simulink model "fuzzy_PI"  (R2021a)
settings: Solver=VariableStepAuto  StartTime=0.0  StopTime=0.05  RelTol=1e-3
libraries: pid_lib x5, spsPermanentMagnetSynchronousMachineLib x2, spsDCVoltageSourceLib x2, spsUniversalBridgeLib x2, simulink x2, eeGeneralControl x1, spspowerguiLib x1, fuzblock x1
settings Model: Creator=lijingze  LastModifiedBy=lijingze

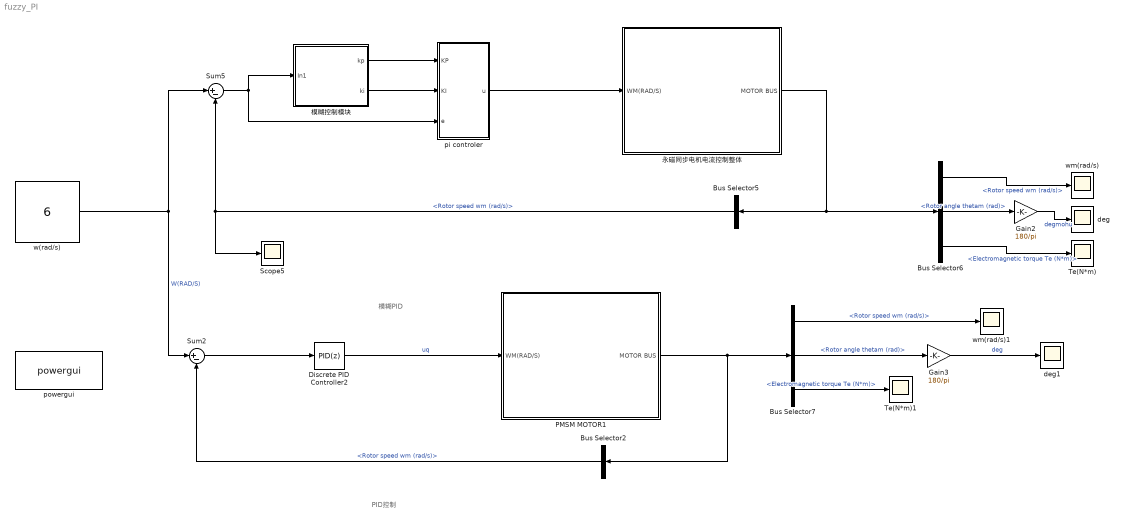
== system fuzzy_PI ==
  note: PID控制
  note: 模糊PID
  Bus Selector2 : BusSelector  OutputSignals=Rotor speed wm (rad/s)
  Bus Selector5 : BusSelector  OutputSignals=Rotor speed wm (rad/s)
  Bus Selector6 : BusSelector  OutputSignals=Rotor speed wm (rad/s),Rotor angle thetam (rad),Electromagnetic torque Te (N*m)
  Bus Selector7 : BusSelector  OutputSignals=Rotor speed wm (rad/s),Rotor angle thetam (rad),Electromagnetic torque Te (N*m)
  Discrete PID Controller2 : pid_lib/PID Controller  Controller=PID  Form=Parallel  TimeDomain=Discrete-time  UseExternalTs=off  SampleTime=-1  IntegratorMethod=Forward Euler  FilterMethod=Forward Euler  ControllerParametersSource=internal  P=40  I=3000  D=0  UseFilter=on  N=100  TunerSelectOption=Transfer Function Based (PID Tuner App)  InitialConditionSource=internal  InitialConditionForIntegrator=0  InitialConditionForFilter=0  DifferentiatorICPrevScaledInput=0  ExternalReset=none  TrackingMode=off  Kt=1  LimitOutput=on  SatLimitsSource=internal  UpperSaturationLimit=100  LowerSaturationLimit=-100  LinearizeAsGain=off  AntiWindupMode=none  Kb=1  POutMin=[]  POutMax=[]  IOutMin=[]  IOutMax=[]  DOutMin=[]  DOutMax=[]  NOutMin=[]  NOutMax=[]  SumOutMin=[]  SumOutMax=[]  SaturationOutMin=[]  SaturationOutMax=[]  PParamMin=[]  PParamMax=[]  IParamMin=[]  IParamMax=[]  DParamMin=[]  DParamMax=[]  NParamMin=[]  NParamMax=[]  KbParamMin=[]  KbParamMax=[]  KtParamMin=[]  KtParamMax=[]  KbOutMin=[]  KbOutMax=[]  KtOutMin=[]  KtOutMax=[]  IntegratorOutMin=[]  IntegratorOutMax=[]  FilterOutMin=[]  FilterOutMax=[]  SumI1OutMin=[]  SumI1OutMax=[]  SumI2OutMin=[]  SumI2OutMax=[]  SumI3OutMin=[]  SumI3OutMax=[]  SumI4OutMin=[]  SumI4OutMax=[]  SumDOutMin=[]  SumDOutMax=[]  DifferentiatorOutMin=[]  DifferentiatorOutMax=[]  FilterDiffOutCoefMin=[]  FilterDiffOutCoefMax=[]  ReciprocalOutMin=[]  ReciprocalOutMax=[]  SumDenOutMin=[]  SumDenOutMax=[]  SumNumOutMin=[]  SumNumOutMax=[]  DivideOutMin=[]  DivideOutMax=[]  UdiffTsProdOutMin=[]  UdiffTsProdOutMax=[]  NTsProdOutMin=[]  NTsProdOutMax=[]  UintegralTsProdOutMin=[]  UintegralTsProdOutMax=[]  UngainTsProdOutMin=[]  UngainTsProdOutMax=[]  IntegratorContinuousStateAttributes=''  IntegratorStateMustResolveToSignalObject=off  IntegratorRTWStateStorageClass=Auto  FilterContinuousStateAttributes=''  FilterStateMustResolveToSignalObject=off  FilterRTWStateStorageClass=Auto  ParallelPVariant=InternalParameters  IdealPVariant=Disabled  IVariant=InternalParameters  DVariant=InternalParameters  IntegratorVariant=Discrete  SatVariant=Enabled  AWVariant=Passthrough  PCopyVariant=Disabled  TRVariant=Disabled  FdbkBlocksVariant=Forward  IdealPFdbkVariant=Disabled  SatFdbkVariant=Disabled  DerivativeFilterVariant=ForwardEulerFilter  NVariant=InternalParameters  NCopyVariant=Disabled  FilterICVariant=InternalICsFilter  IntegratorICVariant=InternalICs  ExternalResetVariant=Disabled  TRSumVariant=Passthrough  SumFdbkVariant=Disabled  SumVariant=Sum_PID  TsampFilterVariant=InternalTs  TsampNgainVariant=Passthrough  TsampIntegralVariant=Passthrough  ExternalSaturationOutDataTypeStr=Inherit: Same as second input
  Gain2 : Gain  Gain=180/pi
  Gain3 : Gain  Gain=180/pi
  PMSM MOTOR1 : Subsystem
  Scope5 : Scope
  Sum2 : Sum  Inputs=|+-
  Sum5 : Sum  Inputs=|+-
  Te(N*m) : Scope
  Te(N*m)1 : Scope
  deg : Scope
  deg1 : Scope
  pi controler : Subsystem
  powergui : spspowerguiLib/powergui  Priority=1  SimulationMode=Discrete  SampleTime=2e-6  frequency=60  Iterations=50  frequencyindice=0  Pbase=100e6  ErrMax=1e-4  UnitsV=kV  UnitsW=MW  buscounter=0  FunctionMessages=off  echomessages=off  EnableUseOfTLC=off  CurrentSourceSwitches=off  DisableSnubberDevices=off  DisableRonSwitches=off  DisableVfSwitches=off  DisplayEquations=off  AutomaticDiscreteSolvers=off  SolverType=Tustin/Backward Euler (TBE)  Interpol=off  ExternalGateDelay=off  methode=off  Ts=100  x0status=blocks  SPID=on  SwTol=0  HookPort=off  NonlinearTolerance=1e-4  nMaxIteration=100  ContinueOnMaxIteration=off  RestoreLinks=warning  ResistiveCurrentMeasurement=off  Frange=[0:2:500]  Ylog=off  Xlog=on  ShowGrid=off  save=off  variable=ZData  structure=0  ZoomFFT=off  StartTime=0.0  cycles=1  DisplayStyle=1  fundamental=60  FreqAxis=off  MaxFrequency=1000  frequencyindicesteady=1  RmsSteady=1  display=off
  w(rad/s) : Constant  Value=6
  wm(rad/s) : Scope
  wm(rad/s)1 : Scope
  模糊控制模块 : Subsystem
  永磁同步电机电流控制整体 : Subsystem
  wires:
  PMSM MOTOR1/1(MOTOR BUS) -> Bus Selector2/1, Bus Selector7/1
  Discrete PID Controller2/1 -> PMSM MOTOR1/1(WM(RAD/S))  "uq"
  永磁同步电机电流控制整体/1(MOTOR BUS) -> Bus Selector5/1, Bus Selector6/1
  pi controler/1(u) -> 永磁同步电机电流控制整体/1(WM(RAD/S))
  Bus Selector6/1 -> wm(rad/s)/1  "<Rotor speed wm (rad/s)>"
  Sum2/1 -> Discrete PID Controller2/1
  Bus Selector6/2 -> Gain2/1  "<Rotor angle thetam (rad)>"
  Bus Selector2/1 -> Sum2/2  "<Rotor speed wm (rad/s)>"
  Bus Selector5/1 -> Scope5/1, Sum5/2  "<Rotor speed wm (rad/s)>"
  Bus Selector6/3 -> Te(N*m)/1  "<Electromagnetic torque Te (N*m)>"
  Gain2/1 -> deg/1  "degmohu"
  Bus Selector7/2 -> Gain3/1  "<Rotor angle thetam (rad)>"
  Sum5/1 -> 模糊控制模块/1(In1), pi controler/3(e)
  w(rad/s)/1 -> Sum2/1, Sum5/1  "W(RAD/S)"
  模糊控制模块/2(ki) -> pi controler/2(KI)
  模糊控制模块/1(kp) -> pi controler/1(KP)
  Bus Selector7/1 -> wm(rad/s)1/1  "<Rotor speed wm (rad/s)>"
  Gain3/1 -> deg1/1  "deg"
  Bus Selector7/3 -> Te(N*m)1/1  "<Electromagnetic torque Te (N*m)>"

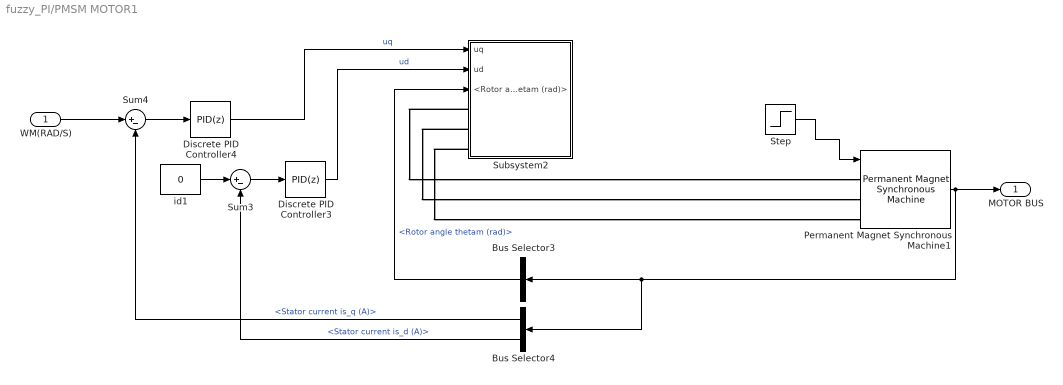
== system fuzzy_PI/PMSM MOTOR1 ==
  WM(RAD/S) : Inport
  Bus Selector3 : BusSelector  OutputSignals=Rotor angle thetam (rad)
  Bus Selector4 : BusSelector  OutputSignals=Stator current is_q (A),Stator current is_d (A)
  Discrete PID Controller3 : pid_lib/PID Controller  Controller=PID  Form=Parallel  TimeDomain=Discrete-time  UseExternalTs=off  SampleTime=-1  IntegratorMethod=Forward Euler  FilterMethod=Forward Euler  ControllerParametersSource=internal  P=50  I=5000  D=0  UseFilter=on  N=100  TunerSelectOption=Transfer Function Based (PID Tuner App)  InitialConditionSource=internal  InitialConditionForIntegrator=0  InitialConditionForFilter=0  DifferentiatorICPrevScaledInput=0  ExternalReset=none  TrackingMode=off  Kt=1  LimitOutput=on  SatLimitsSource=internal  UpperSaturationLimit=100  LowerSaturationLimit=-100  LinearizeAsGain=off  AntiWindupMode=none  Kb=1  POutMin=[]  POutMax=[]  IOutMin=[]  IOutMax=[]  DOutMin=[]  DOutMax=[]  NOutMin=[]  NOutMax=[]  SumOutMin=[]  SumOutMax=[]  SaturationOutMin=[]  SaturationOutMax=[]  PParamMin=[]  PParamMax=[]  IParamMin=[]  IParamMax=[]  DParamMin=[]  DParamMax=[]  NParamMin=[]  NParamMax=[]  KbParamMin=[]  KbParamMax=[]  KtParamMin=[]  KtParamMax=[]  KbOutMin=[]  KbOutMax=[]  KtOutMin=[]  KtOutMax=[]  IntegratorOutMin=[]  IntegratorOutMax=[]  FilterOutMin=[]  FilterOutMax=[]  SumI1OutMin=[]  SumI1OutMax=[]  SumI2OutMin=[]  SumI2OutMax=[]  SumI3OutMin=[]  SumI3OutMax=[]  SumI4OutMin=[]  SumI4OutMax=[]  SumDOutMin=[]  SumDOutMax=[]  DifferentiatorOutMin=[]  DifferentiatorOutMax=[]  FilterDiffOutCoefMin=[]  FilterDiffOutCoefMax=[]  ReciprocalOutMin=[]  ReciprocalOutMax=[]  SumDenOutMin=[]  SumDenOutMax=[]  SumNumOutMin=[]  SumNumOutMax=[]  DivideOutMin=[]  DivideOutMax=[]  UdiffTsProdOutMin=[]  UdiffTsProdOutMax=[]  NTsProdOutMin=[]  NTsProdOutMax=[]  UintegralTsProdOutMin=[]  UintegralTsProdOutMax=[]  UngainTsProdOutMin=[]  UngainTsProdOutMax=[]  IntegratorContinuousStateAttributes=''  IntegratorStateMustResolveToSignalObject=off  IntegratorRTWStateStorageClass=Auto  FilterContinuousStateAttributes=''  FilterStateMustResolveToSignalObject=off  FilterRTWStateStorageClass=Auto  ParallelPVariant=InternalParameters  IdealPVariant=Disabled  IVariant=InternalParameters  DVariant=InternalParameters  IntegratorVariant=Discrete  SatVariant=Enabled  AWVariant=Passthrough  PCopyVariant=Disabled  TRVariant=Disabled  FdbkBlocksVariant=Forward  IdealPFdbkVariant=Disabled  SatFdbkVariant=Disabled  DerivativeFilterVariant=ForwardEulerFilter  NVariant=InternalParameters  NCopyVariant=Disabled  FilterICVariant=InternalICsFilter  IntegratorICVariant=InternalICs  ExternalResetVariant=Disabled  TRSumVariant=Passthrough  SumFdbkVariant=Disabled  SumVariant=Sum_PID  TsampFilterVariant=InternalTs  TsampNgainVariant=Passthrough  TsampIntegralVariant=Passthrough  ExternalSaturationOutDataTypeStr=Inherit: Same as second input
  Discrete PID Controller4 : pid_lib/PID Controller  Controller=PID  Form=Parallel  TimeDomain=Discrete-time  UseExternalTs=off  SampleTime=-1  IntegratorMethod=Forward Euler  FilterMethod=Forward Euler  ControllerParametersSource=internal  P=50  I=5000  D=0  UseFilter=on  N=100  TunerSelectOption=Transfer Function Based (PID Tuner App)  InitialConditionSource=internal  InitialConditionForIntegrator=0  InitialConditionForFilter=0  DifferentiatorICPrevScaledInput=0  ExternalReset=none  TrackingMode=off  Kt=1  LimitOutput=on  SatLimitsSource=internal  UpperSaturationLimit=100  LowerSaturationLimit=-100  LinearizeAsGain=off  AntiWindupMode=none  Kb=1  POutMin=[]  POutMax=[]  IOutMin=[]  IOutMax=[]  DOutMin=[]  DOutMax=[]  NOutMin=[]  NOutMax=[]  SumOutMin=[]  SumOutMax=[]  SaturationOutMin=[]  SaturationOutMax=[]  PParamMin=[]  PParamMax=[]  IParamMin=[]  IParamMax=[]  DParamMin=[]  DParamMax=[]  NParamMin=[]  NParamMax=[]  KbParamMin=[]  KbParamMax=[]  KtParamMin=[]  KtParamMax=[]  KbOutMin=[]  KbOutMax=[]  KtOutMin=[]  KtOutMax=[]  IntegratorOutMin=[]  IntegratorOutMax=[]  FilterOutMin=[]  FilterOutMax=[]  SumI1OutMin=[]  SumI1OutMax=[]  SumI2OutMin=[]  SumI2OutMax=[]  SumI3OutMin=[]  SumI3OutMax=[]  SumI4OutMin=[]  SumI4OutMax=[]  SumDOutMin=[]  SumDOutMax=[]  DifferentiatorOutMin=[]  DifferentiatorOutMax=[]  FilterDiffOutCoefMin=[]  FilterDiffOutCoefMax=[]  ReciprocalOutMin=[]  ReciprocalOutMax=[]  SumDenOutMin=[]  SumDenOutMax=[]  SumNumOutMin=[]  SumNumOutMax=[]  DivideOutMin=[]  DivideOutMax=[]  UdiffTsProdOutMin=[]  UdiffTsProdOutMax=[]  NTsProdOutMin=[]  NTsProdOutMax=[]  UintegralTsProdOutMin=[]  UintegralTsProdOutMax=[]  UngainTsProdOutMin=[]  UngainTsProdOutMax=[]  IntegratorContinuousStateAttributes=''  IntegratorStateMustResolveToSignalObject=off  IntegratorRTWStateStorageClass=Auto  FilterContinuousStateAttributes=''  FilterStateMustResolveToSignalObject=off  FilterRTWStateStorageClass=Auto  ParallelPVariant=InternalParameters  IdealPVariant=Disabled  IVariant=InternalParameters  DVariant=InternalParameters  IntegratorVariant=Discrete  SatVariant=Enabled  AWVariant=Passthrough  PCopyVariant=Disabled  TRVariant=Disabled  FdbkBlocksVariant=Forward  IdealPFdbkVariant=Disabled  SatFdbkVariant=Disabled  DerivativeFilterVariant=ForwardEulerFilter  NVariant=InternalParameters  NCopyVariant=Disabled  FilterICVariant=InternalICsFilter  IntegratorICVariant=InternalICs  ExternalResetVariant=Disabled  TRSumVariant=Passthrough  SumFdbkVariant=Disabled  SumVariant=Sum_PID  TsampFilterVariant=InternalTs  TsampNgainVariant=Passthrough  TsampIntegralVariant=Passthrough  ExternalSaturationOutDataTypeStr=Inherit: Same as second input
  Permanent Magnet Synchronous Machine1 : spsPermanentMagnetSynchronousMachineLib/Permanent Magnet Synchronous Machine  NbPhases=3  FluxDistribution=Sinusoidal  RotorType=Round  MechanicalLoad=Torque Tm  PresetModel=No  ShowDetailedParameters=on  MeasurementBus=off  Resistance=0.0485  Inductance=8.5e-3  dqInductances=[8.5e-3,8.5e-3]  La=0.000395  MachineConstant=Flux linkage established by magnets (V.s)  Flux=0.1194  VoltageCst=21.6568  TorqueCst=0.1791  Flat=120  Mechanical=[0.0027 0.04924 1 0]  PolePairs=4  InitialConditions=[0,0, 0,0]  InitialConditions5ph=[0 0 0 0 0 0]  RefAngle=Aligned with phase A axis (original Park)  IterativeDiscreteModel=Trapezoidal non iterative  TsBlock=-1  TsPowergui=0
  Step : Step  Time=0.025  Before=5  After=10  SampleTime=0.025
  Subsystem2 : Subsystem
  Sum3 : Sum  Inputs=|+-
  Sum4 : Sum  Inputs=|+-
  id1 : Constant  Value=0
  MOTOR BUS : Outport
  wires:
  Discrete PID Controller3/1 -> Subsystem2/2(ud)  "ud"
  Bus Selector3/1 -> Subsystem2/3(<Rotor angle thetam (rad)>)  "<Rotor angle thetam (rad)>"
  Sum4/1 -> Discrete PID Controller4/1
  Permanent Magnet Synchronous Machine1/1 -> Bus Selector4/1, Bus Selector3/1, MOTOR BUS/1
  id1/1 -> Sum3/1
  Bus Selector4/2 -> Sum3/2  "<Stator current is_d (A)>"
  Discrete PID Controller4/1 -> Subsystem2/1(uq)  "uq"
  Sum3/1 -> Discrete PID Controller3/1
  Bus Selector4/1 -> Sum4/2  "<Stator current is_q (A)>"
  Step/1 -> Permanent Magnet Synchronous Machine1/1
  WM(RAD/S)/1 -> Sum4/1
  connections:
  Subsystem2/LConn3 -- Permanent Magnet Synchronous Machine1/LConn3
  Subsystem2/LConn2 -- Permanent Magnet Synchronous Machine1/LConn2
  Subsystem2/LConn1 -- Permanent Magnet Synchronous Machine1/LConn1

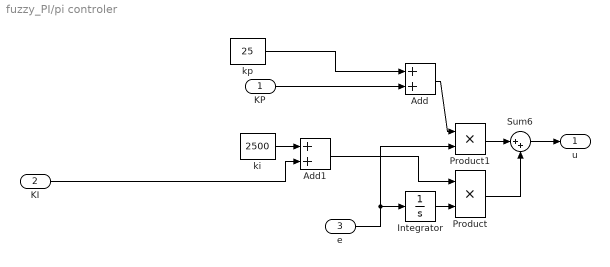
== system fuzzy_PI/pi controler ==
  KP : Inport
  KI : Inport  Port=2
  e : Inport  Port=3
  Add : Sum
  Add1 : Sum
  Integrator : Integrator
  Product : Product
  Product1 : Product
  Sum6 : Sum  Inputs=|++
  ki : Constant  Value=2500
  kp : Constant  Value=25
  u : Outport
  wires:
  Integrator/1 -> Product/2
  e/1 -> Product1/2, Integrator/1
  Product1/1 -> Sum6/1
  Product/1 -> Sum6/2
  Sum6/1 -> u/1
  KP/1 -> Add/2
  kp/1 -> Add/1
  Add/1 -> Product1/1
  ki/1 -> Add1/1
  KI/1 -> Add1/2
  Add1/1 -> Product/1

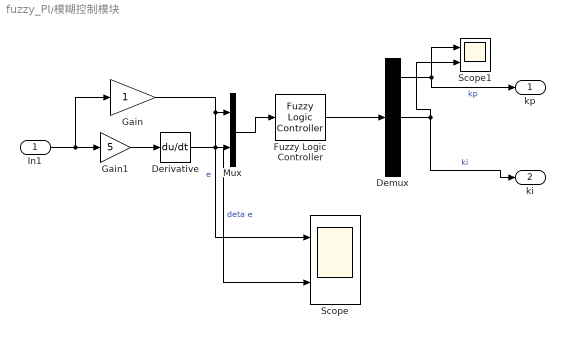
== system fuzzy_PI/模糊控制模块 ==
  In1 : Inport
  Demux : Demux  Outputs=3
  Derivative : Derivative
  Fuzzy Logic Controller : fuzblock/Fuzzy Logic  Controller  FIS=fuzzy_pid  OutputSampleNumber=101  DataType=double  FuzzifiedInputs=off  RuleFiringStrengths=off  RuleOutputs=off  AggregatedOutputs=off  SimulateUsing=Code generation  OutOfRangeInputValueMessage=warning  NoRuleFiredMessage=warning  EmptyOutputFuzzySetMessage=warning
  Gain : Gain
  Gain1 : Gain  Gain=5
  Mux : Mux  Inputs=2
  Scope : Scope  NumInputPorts=2
  Scope1 : Scope  NumInputPorts=2
  kp : Outport
  ki : Outport  Port=2
  wires:
  In1/1 -> Gain/1, Gain1/1
  Mux/1 -> Fuzzy Logic Controller/1
  Gain/1 -> Scope/1, Mux/1  "e"
  Gain1/1 -> Derivative/1
  Derivative/1 -> Scope/2, Mux/2  "deta e"
  Fuzzy Logic Controller/1 -> Demux/1
  Demux/1 -> kp/1, Scope1/1  "kp"
  Demux/2 -> ki/1, Scope1/2  "ki"

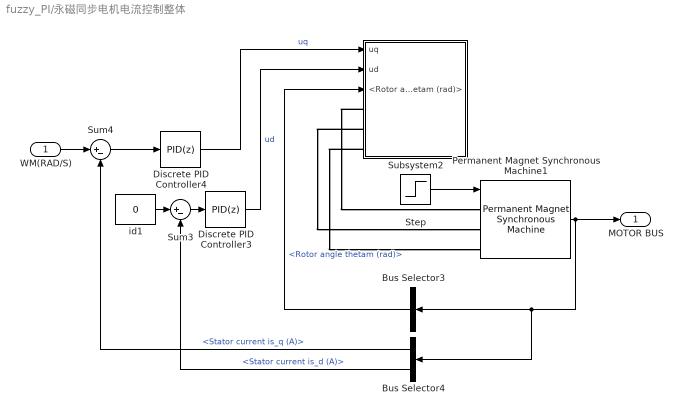
== system fuzzy_PI/永磁同步电机电流控制整体 ==
  WM(RAD/S) : Inport
  Bus Selector3 : BusSelector  OutputSignals=Rotor angle thetam (rad)
  Bus Selector4 : BusSelector  OutputSignals=Stator current is_q (A),Stator current is_d (A)
  Discrete PID Controller3 : pid_lib/PID Controller  Controller=PID  Form=Parallel  TimeDomain=Discrete-time  UseExternalTs=off  SampleTime=-1  IntegratorMethod=Forward Euler  FilterMethod=Forward Euler  ControllerParametersSource=internal  P=50  I=5000  D=0  UseFilter=on  N=100  TunerSelectOption=Transfer Function Based (PID Tuner App)  InitialConditionSource=internal  InitialConditionForIntegrator=0  InitialConditionForFilter=0  DifferentiatorICPrevScaledInput=0  ExternalReset=none  TrackingMode=off  Kt=1  LimitOutput=on  SatLimitsSource=internal  UpperSaturationLimit=100  LowerSaturationLimit=-100  LinearizeAsGain=off  AntiWindupMode=none  Kb=1  POutMin=[]  POutMax=[]  IOutMin=[]  IOutMax=[]  DOutMin=[]  DOutMax=[]  NOutMin=[]  NOutMax=[]  SumOutMin=[]  SumOutMax=[]  SaturationOutMin=[]  SaturationOutMax=[]  PParamMin=[]  PParamMax=[]  IParamMin=[]  IParamMax=[]  DParamMin=[]  DParamMax=[]  NParamMin=[]  NParamMax=[]  KbParamMin=[]  KbParamMax=[]  KtParamMin=[]  KtParamMax=[]  KbOutMin=[]  KbOutMax=[]  KtOutMin=[]  KtOutMax=[]  IntegratorOutMin=[]  IntegratorOutMax=[]  FilterOutMin=[]  FilterOutMax=[]  SumI1OutMin=[]  SumI1OutMax=[]  SumI2OutMin=[]  SumI2OutMax=[]  SumI3OutMin=[]  SumI3OutMax=[]  SumI4OutMin=[]  SumI4OutMax=[]  SumDOutMin=[]  SumDOutMax=[]  DifferentiatorOutMin=[]  DifferentiatorOutMax=[]  FilterDiffOutCoefMin=[]  FilterDiffOutCoefMax=[]  ReciprocalOutMin=[]  ReciprocalOutMax=[]  SumDenOutMin=[]  SumDenOutMax=[]  SumNumOutMin=[]  SumNumOutMax=[]  DivideOutMin=[]  DivideOutMax=[]  UdiffTsProdOutMin=[]  UdiffTsProdOutMax=[]  NTsProdOutMin=[]  NTsProdOutMax=[]  UintegralTsProdOutMin=[]  UintegralTsProdOutMax=[]  UngainTsProdOutMin=[]  UngainTsProdOutMax=[]  IntegratorContinuousStateAttributes=''  IntegratorStateMustResolveToSignalObject=off  IntegratorRTWStateStorageClass=Auto  FilterContinuousStateAttributes=''  FilterStateMustResolveToSignalObject=off  FilterRTWStateStorageClass=Auto  ParallelPVariant=InternalParameters  IdealPVariant=Disabled  IVariant=InternalParameters  DVariant=InternalParameters  IntegratorVariant=Discrete  SatVariant=Enabled  AWVariant=Passthrough  PCopyVariant=Disabled  TRVariant=Disabled  FdbkBlocksVariant=Forward  IdealPFdbkVariant=Disabled  SatFdbkVariant=Disabled  DerivativeFilterVariant=ForwardEulerFilter  NVariant=InternalParameters  NCopyVariant=Disabled  FilterICVariant=InternalICsFilter  IntegratorICVariant=InternalICs  ExternalResetVariant=Disabled  TRSumVariant=Passthrough  SumFdbkVariant=Disabled  SumVariant=Sum_PID  TsampFilterVariant=InternalTs  TsampNgainVariant=Passthrough  TsampIntegralVariant=Passthrough  ExternalSaturationOutDataTypeStr=Inherit: Same as second input
  Discrete PID Controller4 : pid_lib/PID Controller  Controller=PID  Form=Parallel  TimeDomain=Discrete-time  UseExternalTs=off  SampleTime=-1  IntegratorMethod=Forward Euler  FilterMethod=Forward Euler  ControllerParametersSource=internal  P=50  I=5000  D=0  UseFilter=on  N=100  TunerSelectOption=Transfer Function Based (PID Tuner App)  InitialConditionSource=internal  InitialConditionForIntegrator=0  InitialConditionForFilter=0  DifferentiatorICPrevScaledInput=0  ExternalReset=none  TrackingMode=off  Kt=1  LimitOutput=on  SatLimitsSource=internal  UpperSaturationLimit=100  LowerSaturationLimit=-100  LinearizeAsGain=off  AntiWindupMode=none  Kb=1  POutMin=[]  POutMax=[]  IOutMin=[]  IOutMax=[]  DOutMin=[]  DOutMax=[]  NOutMin=[]  NOutMax=[]  SumOutMin=[]  SumOutMax=[]  SaturationOutMin=[]  SaturationOutMax=[]  PParamMin=[]  PParamMax=[]  IParamMin=[]  IParamMax=[]  DParamMin=[]  DParamMax=[]  NParamMin=[]  NParamMax=[]  KbParamMin=[]  KbParamMax=[]  KtParamMin=[]  KtParamMax=[]  KbOutMin=[]  KbOutMax=[]  KtOutMin=[]  KtOutMax=[]  IntegratorOutMin=[]  IntegratorOutMax=[]  FilterOutMin=[]  FilterOutMax=[]  SumI1OutMin=[]  SumI1OutMax=[]  SumI2OutMin=[]  SumI2OutMax=[]  SumI3OutMin=[]  SumI3OutMax=[]  SumI4OutMin=[]  SumI4OutMax=[]  SumDOutMin=[]  SumDOutMax=[]  DifferentiatorOutMin=[]  DifferentiatorOutMax=[]  FilterDiffOutCoefMin=[]  FilterDiffOutCoefMax=[]  ReciprocalOutMin=[]  ReciprocalOutMax=[]  SumDenOutMin=[]  SumDenOutMax=[]  SumNumOutMin=[]  SumNumOutMax=[]  DivideOutMin=[]  DivideOutMax=[]  UdiffTsProdOutMin=[]  UdiffTsProdOutMax=[]  NTsProdOutMin=[]  NTsProdOutMax=[]  UintegralTsProdOutMin=[]  UintegralTsProdOutMax=[]  UngainTsProdOutMin=[]  UngainTsProdOutMax=[]  IntegratorContinuousStateAttributes=''  IntegratorStateMustResolveToSignalObject=off  IntegratorRTWStateStorageClass=Auto  FilterContinuousStateAttributes=''  FilterStateMustResolveToSignalObject=off  FilterRTWStateStorageClass=Auto  ParallelPVariant=InternalParameters  IdealPVariant=Disabled  IVariant=InternalParameters  DVariant=InternalParameters  IntegratorVariant=Discrete  SatVariant=Enabled  AWVariant=Passthrough  PCopyVariant=Disabled  TRVariant=Disabled  FdbkBlocksVariant=Forward  IdealPFdbkVariant=Disabled  SatFdbkVariant=Disabled  DerivativeFilterVariant=ForwardEulerFilter  NVariant=InternalParameters  NCopyVariant=Disabled  FilterICVariant=InternalICsFilter  IntegratorICVariant=InternalICs  ExternalResetVariant=Disabled  TRSumVariant=Passthrough  SumFdbkVariant=Disabled  SumVariant=Sum_PID  TsampFilterVariant=InternalTs  TsampNgainVariant=Passthrough  TsampIntegralVariant=Passthrough  ExternalSaturationOutDataTypeStr=Inherit: Same as second input
  Permanent Magnet Synchronous Machine1 : spsPermanentMagnetSynchronousMachineLib/Permanent Magnet Synchronous Machine  NbPhases=3  FluxDistribution=Sinusoidal  RotorType=Round  MechanicalLoad=Torque Tm  PresetModel=No  ShowDetailedParameters=on  MeasurementBus=off  Resistance=0.0485  Inductance=8.5e-3  dqInductances=[8.5e-3,8.5e-3]  La=0.000395  MachineConstant=Flux linkage established by magnets (V.s)  Flux=0.1194  VoltageCst=21.6568  TorqueCst=0.1791  Flat=120  Mechanical=[0.0027 0.04924 1 0]  PolePairs=4  InitialConditions=[0,0, 0,0]  InitialConditions5ph=[0 0 0 0 0 0]  RefAngle=Aligned with phase A axis (original Park)  IterativeDiscreteModel=Trapezoidal non iterative  TsBlock=-1  TsPowergui=0
  Step : Step  Time=0.025  Before=5  After=10  SampleTime=0.025
  Subsystem2 : Subsystem
  Sum3 : Sum  Inputs=|+-
  Sum4 : Sum  Inputs=|+-
  id1 : Constant  Value=0
  MOTOR BUS : Outport
  wires:
  Discrete PID Controller3/1 -> Subsystem2/2(ud)  "ud"
  Bus Selector3/1 -> Subsystem2/3(<Rotor angle thetam (rad)>)  "<Rotor angle thetam (rad)>"
  Sum4/1 -> Discrete PID Controller4/1
  Permanent Magnet Synchronous Machine1/1 -> Bus Selector4/1, Bus Selector3/1, MOTOR BUS/1
  id1/1 -> Sum3/1
  Bus Selector4/2 -> Sum3/2  "<Stator current is_d (A)>"
  Discrete PID Controller4/1 -> Subsystem2/1(uq)  "uq"
  Sum3/1 -> Discrete PID Controller3/1
  Bus Selector4/1 -> Sum4/2  "<Stator current is_q (A)>"
  WM(RAD/S)/1 -> Sum4/1
  Step/1 -> Permanent Magnet Synchronous Machine1/1
  connections:
  Subsystem2/LConn3 -- Permanent Magnet Synchronous Machine1/LConn3
  Subsystem2/LConn2 -- Permanent Magnet Synchronous Machine1/LConn2
  Subsystem2/LConn1 -- Permanent Magnet Synchronous Machine1/LConn1

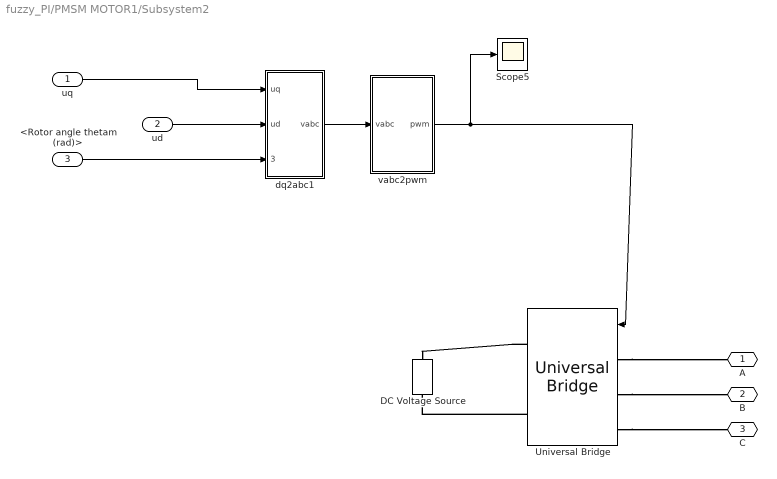
== system fuzzy_PI/PMSM MOTOR1/Subsystem2 ==
  uq : Inport
  ud : Inport  Port=2
  <Rotor angle thetam (rad)> : Inport  Port=3
  DC Voltage Source : spsDCVoltageSourceLib/DC Voltage Source  Amplitude=100  Measurements=None
  Scope5 : Scope
  Universal Bridge : spsUniversalBridgeLib/Universal Bridge  Arms=3  SnubberResistance=1e5  SnubberCapacitance=inf  Device=MOSFET / Diodes  Ron=1e-3  Lon=0  ForwardVoltages="[  0  0  ]"  ForwardVoltage=0  GTOparameters=[ 10e-6 , 20e-6 ]  IGBTparameters=[ 1e-6 , 2e-6 ]  Measurements=None  Measurements_2=None  converterType=Rectifier
  dq2abc1 : Subsystem
  vabc2pwm : Subsystem
  A : PMIOPort  Side=Left
  B : PMIOPort  Port=2  Side=Left
  C : PMIOPort  Port=3  Side=Left
  wires:
  uq/1 -> dq2abc1/1(uq)
  <Rotor angle thetam (rad)>/1 -> dq2abc1/3(" theta")
  vabc2pwm/1(pwm) -> Scope5/1, Universal Bridge/1
  ud/1 -> dq2abc1/2(ud)
  dq2abc1/1(vabc) -> vabc2pwm/1(vabc)
  connections:
  Universal Bridge/LConn2 -- B/RConn1
  Universal Bridge/RConn1 -- DC Voltage Source/RConn1
  Universal Bridge/RConn2 -- DC Voltage Source/LConn1
  Universal Bridge/LConn1 -- A/RConn1
  Universal Bridge/LConn3 -- C/RConn1

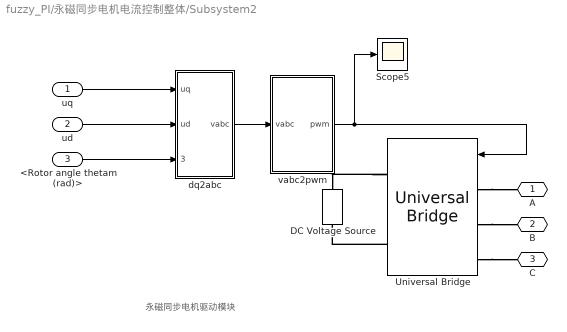
== system fuzzy_PI/永磁同步电机电流控制整体/Subsystem2 ==
  note: 永磁同步电机驱动模块
  uq : Inport
  ud : Inport  Port=2
  <Rotor angle thetam (rad)> : Inport  Port=3
  DC Voltage Source : spsDCVoltageSourceLib/DC Voltage Source  Amplitude=100  Measurements=None
  Scope5 : Scope
  Universal Bridge : spsUniversalBridgeLib/Universal Bridge  Arms=3  SnubberResistance=1e5  SnubberCapacitance=inf  Device=MOSFET / Diodes  Ron=1e-3  Lon=0  ForwardVoltages="[  0  0  ]"  ForwardVoltage=0  GTOparameters=[ 10e-6 , 20e-6 ]  IGBTparameters=[ 1e-6 , 2e-6 ]  Measurements=None  Measurements_2=None  converterType=Rectifier
  dq2abc : Subsystem
  vabc2pwm : Subsystem
  A : PMIOPort  Side=Left
  B : PMIOPort  Port=2  Side=Left
  C : PMIOPort  Port=3  Side=Left
  wires:
  uq/1 -> dq2abc/1(uq)
  <Rotor angle thetam (rad)>/1 -> dq2abc/3(" theta")
  vabc2pwm/1(pwm) -> Universal Bridge/1, Scope5/1
  ud/1 -> dq2abc/2(ud)
  dq2abc/1(vabc) -> vabc2pwm/1(vabc)
  connections:
  Universal Bridge/LConn2 -- B/RConn1
  Universal Bridge/RConn1 -- DC Voltage Source/RConn1
  Universal Bridge/RConn2 -- DC Voltage Source/LConn1
  Universal Bridge/LConn1 -- A/RConn1
  Universal Bridge/LConn3 -- C/RConn1

== system fuzzy_PI/PMSM MOTOR1/Subsystem2/dq2abc1 ==
  uq : Inport
  ud : Inport  Port=2
  " theta" : Inport  Port=3
  Mux : Mux  Inputs=3
  Scope1 : Scope
  Subsystem : Subsystem
  Subsystem1 : Subsystem
  Subsystem2 : Subsystem
  vabc : Outport
  wires:
  ud/1 -> Subsystem/2(ud), Subsystem2/2(ud), Subsystem1/2(ud)
  uq/1 -> Subsystem2/1(uq), Subsystem1/1(uq), Subsystem/1(uq)
  " theta"/1 -> Subsystem2/3(" theta"), Subsystem1/3(" theta"), Subsystem/3(" theta")
  Subsystem/1(ua) -> Mux/1
  Mux/1 -> Scope1/1, vabc/1
  Subsystem2/1(ua) -> Mux/3
  Subsystem1/1(ua) -> Mux/2

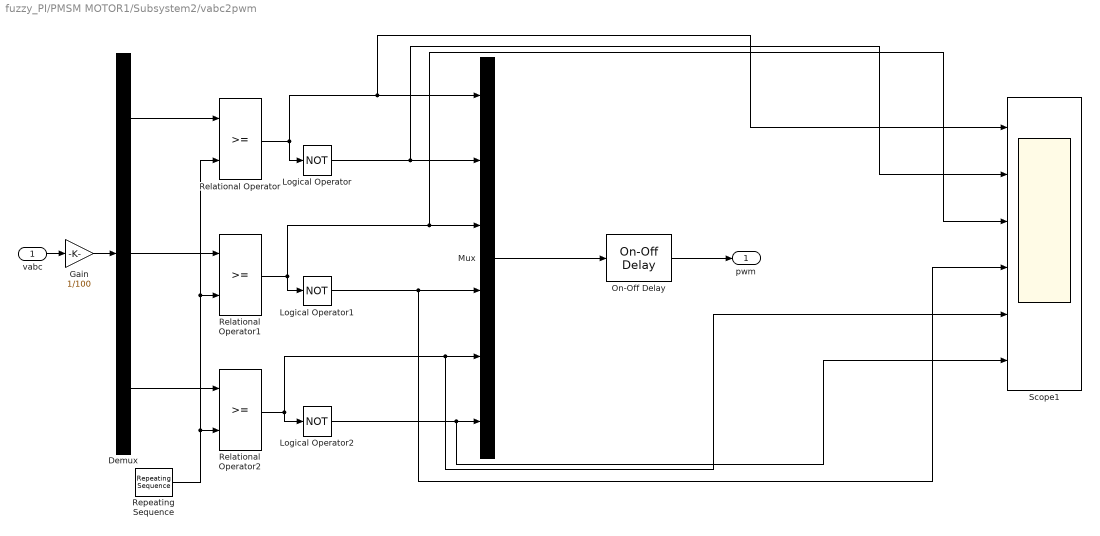
== system fuzzy_PI/PMSM MOTOR1/Subsystem2/vabc2pwm ==
  vabc : Inport
  Demux : Demux  Outputs=3
  Gain : Gain  Gain=1/100
  Logical Operator : Logic  Operator=NOT  AllPortsSameDT=off  OutDataTypeStr=boolean
  Logical Operator1 : Logic  Operator=NOT  AllPortsSameDT=off  OutDataTypeStr=boolean
  Logical Operator2 : Logic  Operator=NOT  AllPortsSameDT=off  OutDataTypeStr=boolean
  Mux : Mux  Inputs=6
  On-Off Delay : eeGeneralControl/On-Off Delay  LabelModeActiveChoice=Discrete  Td_on=2e-6  Td_off=0  IC=0  Ts=2e-6
      settings: SourceProductBaseCode=PS
  Relational Operator : RelationalOperator  OutDataTypeStr=boolean  RndMeth=Simplest
  Relational Operator1 : RelationalOperator  OutDataTypeStr=boolean  RndMeth=Simplest
  Relational Operator2 : RelationalOperator  OutDataTypeStr=boolean  RndMeth=Simplest
  Repeating Sequence : simulink/Sources/Repeating Sequence  rep_seq_t=[0 0.0001]  rep_seq_y=[-1 1]
  Scope1 : Scope  NumInputPorts=6
  pwm : Outport
  wires:
  Repeating Sequence/1 -> Relational Operator/2, Relational Operator1/2, Relational Operator2/2
  Demux/1 -> Relational Operator/1
  Logical Operator/1 -> Scope1/2, Mux/2
  Relational Operator/1 -> Scope1/1, Mux/1, Logical Operator/1
  Demux/3 -> Relational Operator2/1
  Demux/2 -> Relational Operator1/1
  Relational Operator1/1 -> Scope1/3, Mux/3, Logical Operator1/1
  Relational Operator2/1 -> Scope1/5, Mux/5, Logical Operator2/1
  Logical Operator2/1 -> Scope1/6, Mux/6
  Logical Operator1/1 -> Scope1/4, Mux/4
  vabc/1 -> Gain/1
  Gain/1 -> Demux/1
  Mux/1 -> On-Off Delay/1
  On-Off Delay/1 -> pwm/1

== system fuzzy_PI/永磁同步电机电流控制整体/Subsystem2/dq2abc ==
  uq : Inport
  ud : Inport  Port=2
  " theta" : Inport  Port=3
  Mux : Mux  Inputs=3
  Scope1 : Scope
  Subsystem : Subsystem
  Subsystem1 : Subsystem
  Subsystem2 : Subsystem
  vabc : Outport
  wires:
  ud/1 -> Subsystem/2(ud), Subsystem2/2(ud), Subsystem1/2(ud)
  uq/1 -> Subsystem2/1(uq), Subsystem1/1(uq), Subsystem/1(uq)
  " theta"/1 -> Subsystem2/3(" theta"), Subsystem1/3(" theta"), Subsystem/3(" theta")
  Subsystem/1(ua) -> Mux/1
  Mux/1 -> Scope1/1, vabc/1
  Subsystem2/1(ua) -> Mux/3
  Subsystem1/1(ua) -> Mux/2

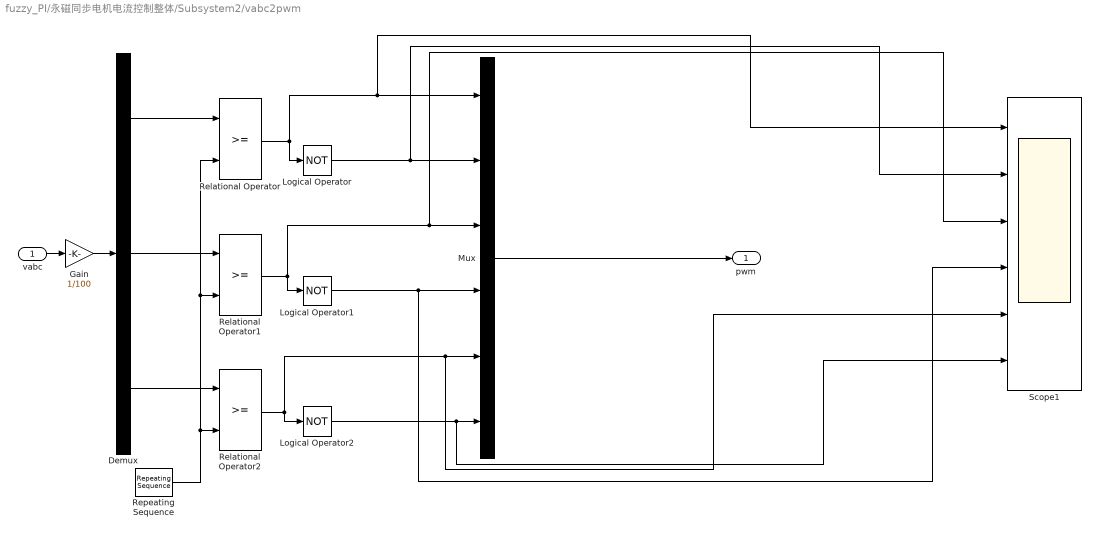
== system fuzzy_PI/永磁同步电机电流控制整体/Subsystem2/vabc2pwm ==
  vabc : Inport
  Demux : Demux  Outputs=3
  Gain : Gain  Gain=1/100
  Logical Operator : Logic  Operator=NOT  AllPortsSameDT=off  OutDataTypeStr=boolean
  Logical Operator1 : Logic  Operator=NOT  AllPortsSameDT=off  OutDataTypeStr=boolean
  Logical Operator2 : Logic  Operator=NOT  AllPortsSameDT=off  OutDataTypeStr=boolean
  Mux : Mux  Inputs=6
  Relational Operator : RelationalOperator  OutDataTypeStr=boolean  RndMeth=Simplest
  Relational Operator1 : RelationalOperator  OutDataTypeStr=boolean  RndMeth=Simplest
  Relational Operator2 : RelationalOperator  OutDataTypeStr=boolean  RndMeth=Simplest
  Repeating Sequence : simulink/Sources/Repeating Sequence  rep_seq_t=[0 0.0001]  rep_seq_y=[-1 1]
  Scope1 : Scope  NumInputPorts=6
  pwm : Outport
  wires:
  Repeating Sequence/1 -> Relational Operator/2, Relational Operator1/2, Relational Operator2/2
  Demux/1 -> Relational Operator/1
  Logical Operator/1 -> Scope1/2, Mux/2
  Relational Operator/1 -> Scope1/1, Mux/1, Logical Operator/1
  Demux/3 -> Relational Operator2/1
  Demux/2 -> Relational Operator1/1
  Relational Operator1/1 -> Scope1/3, Mux/3, Logical Operator1/1
  Relational Operator2/1 -> Scope1/5, Mux/5, Logical Operator2/1
  Logical Operator2/1 -> Scope1/6, Mux/6
  Logical Operator1/1 -> Scope1/4, Mux/4
  vabc/1 -> Gain/1
  Gain/1 -> Demux/1
  Mux/1 -> pwm/1

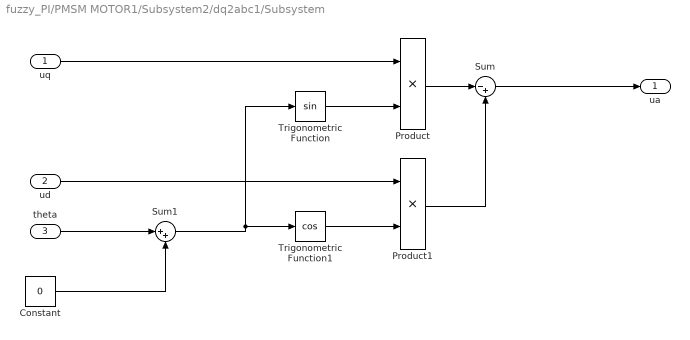
== system fuzzy_PI/PMSM MOTOR1/Subsystem2/dq2abc1/Subsystem ==
  uq : Inport
  ud : Inport  Port=2
  " theta" : Inport  Port=3
  Constant : Constant  Value=0
  Product : Product
  Product1 : Product
  Sum : Sum  Inputs=|-+
  Sum1 : Sum  Inputs=|++
  Trigonometric Function : Trigonometry
  Trigonometric Function1 : Trigonometry  Operator=cos
  ua : Outport
  wires:
  Sum/1 -> ua/1
  Product1/1 -> Sum/2
  ud/1 -> Product1/1
  uq/1 -> Product/1
  Trigonometric Function/1 -> Product/2
  Product/1 -> Sum/1
  Trigonometric Function1/1 -> Product1/2
  " theta"/1 -> Sum1/1
  Sum1/1 -> Trigonometric Function/1, Trigonometric Function1/1
  Constant/1 -> Sum1/2

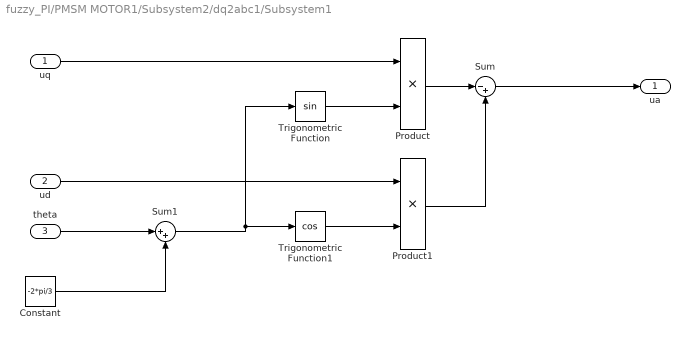
== system fuzzy_PI/PMSM MOTOR1/Subsystem2/dq2abc1/Subsystem1 ==
  uq : Inport
  ud : Inport  Port=2
  " theta" : Inport  Port=3
  Constant : Constant  Value=-2*pi/3
  Product : Product
  Product1 : Product
  Sum : Sum  Inputs=|-+
  Sum1 : Sum  Inputs=|++
  Trigonometric Function : Trigonometry
  Trigonometric Function1 : Trigonometry  Operator=cos
  ua : Outport
  wires:
  Sum/1 -> ua/1
  Product1/1 -> Sum/2
  ud/1 -> Product1/1
  uq/1 -> Product/1
  Trigonometric Function/1 -> Product/2
  Product/1 -> Sum/1
  Trigonometric Function1/1 -> Product1/2
  " theta"/1 -> Sum1/1
  Sum1/1 -> Trigonometric Function/1, Trigonometric Function1/1
  Constant/1 -> Sum1/2

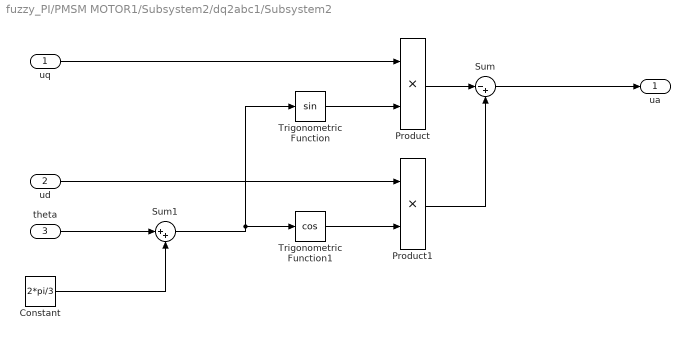
== system fuzzy_PI/PMSM MOTOR1/Subsystem2/dq2abc1/Subsystem2 ==
  uq : Inport
  ud : Inport  Port=2
  " theta" : Inport  Port=3
  Constant : Constant  Value=2*pi/3
  Product : Product
  Product1 : Product
  Sum : Sum  Inputs=|-+
  Sum1 : Sum  Inputs=|++
  Trigonometric Function : Trigonometry
  Trigonometric Function1 : Trigonometry  Operator=cos
  ua : Outport
  wires:
  Sum/1 -> ua/1
  Product1/1 -> Sum/2
  ud/1 -> Product1/1
  uq/1 -> Product/1
  Trigonometric Function/1 -> Product/2
  Product/1 -> Sum/1
  Trigonometric Function1/1 -> Product1/2
  " theta"/1 -> Sum1/1
  Sum1/1 -> Trigonometric Function/1, Trigonometric Function1/1
  Constant/1 -> Sum1/2

== system fuzzy_PI/永磁同步电机电流控制整体/Subsystem2/dq2abc/Subsystem ==
  uq : Inport
  ud : Inport  Port=2
  " theta" : Inport  Port=3
  Constant : Constant  Value=0
  Product : Product
  Product1 : Product
  Sum : Sum  Inputs=|-+
  Sum1 : Sum  Inputs=|++
  Trigonometric Function : Trigonometry
  Trigonometric Function1 : Trigonometry  Operator=cos
  ua : Outport
  wires:
  Sum/1 -> ua/1
  Product1/1 -> Sum/2
  ud/1 -> Product1/1
  uq/1 -> Product/1
  Trigonometric Function/1 -> Product/2
  Product/1 -> Sum/1
  Trigonometric Function1/1 -> Product1/2
  " theta"/1 -> Sum1/1
  Sum1/1 -> Trigonometric Function/1, Trigonometric Function1/1
  Constant/1 -> Sum1/2

== system fuzzy_PI/永磁同步电机电流控制整体/Subsystem2/dq2abc/Subsystem1 ==
  uq : Inport
  ud : Inport  Port=2
  " theta" : Inport  Port=3
  Constant : Constant  Value=-2*pi/3
  Product : Product
  Product1 : Product
  Sum : Sum  Inputs=|-+
  Sum1 : Sum  Inputs=|++
  Trigonometric Function : Trigonometry
  Trigonometric Function1 : Trigonometry  Operator=cos
  ua : Outport
  wires:
  Sum/1 -> ua/1
  Product1/1 -> Sum/2
  ud/1 -> Product1/1
  uq/1 -> Product/1
  Trigonometric Function/1 -> Product/2
  Product/1 -> Sum/1
  Trigonometric Function1/1 -> Product1/2
  " theta"/1 -> Sum1/1
  Sum1/1 -> Trigonometric Function/1, Trigonometric Function1/1
  Constant/1 -> Sum1/2

== system fuzzy_PI/永磁同步电机电流控制整体/Subsystem2/dq2abc/Subsystem2 ==
  uq : Inport
  ud : Inport  Port=2
  " theta" : Inport  Port=3
  Constant : Constant  Value=2*pi/3
  Product : Product
  Product1 : Product
  Sum : Sum  Inputs=|-+
  Sum1 : Sum  Inputs=|++
  Trigonometric Function : Trigonometry
  Trigonometric Function1 : Trigonometry  Operator=cos
  ua : Outport
  wires:
  Sum/1 -> ua/1
  Product1/1 -> Sum/2
  ud/1 -> Product1/1
  uq/1 -> Product/1
  Trigonometric Function/1 -> Product/2
  Product/1 -> Sum/1
  Trigonometric Function1/1 -> Product1/2
  " theta"/1 -> Sum1/1
  Sum1/1 -> Trigonometric Function/1, Trigonometric Function1/1
  Constant/1 -> Sum1/2
